simulink model "RigidbodyMPCCurvePathTracking"  (Simulink 9.3)
settings: Solver=ode45  StartTime=0.0  StopTime=38  FixedStep=0.01  RelTol=1e-3  EnableMultiTasking=on
libraries: Solver_SF x1
settings Model: Creator=xuwei  LastModifiedBy=梁秀华
settings DataIOCC: LimitDataPoints=on
settings OptimizationCC: ExpressionDepthLimit=2147483647
settings DebuggingCC: SolverPrmCheckMsg=warning  StateNameClashWarn=warning
settings GRTTargetCC: GeneratePreprocessorConditionals=Disable all

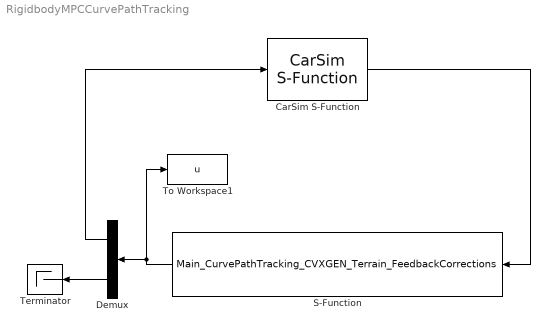
== system RigidbodyMPCCurvePathTracking ==
  CarSim S-Function : Solver_SF/CarSim S-Function  Priority=1  SIMFILE=simfile.sim
  Demux : Demux  Outputs=[1 14]
  S-Function : S-Function  FunctionName=Main_CurvePathTracking_CVXGEN_Terrain_FeedbackCorrections  SFunctionDeploymentMode=off  EnableBusSupport=off
  Terminator : Terminator
  To Workspace1 : ToWorkspace  VariableName=u  SaveFormat=Structure  SampleTime=-1
  wires:
  CarSim S-Function/1 -> S-Function/1
  S-Function/1 -> Demux/1, To Workspace1/1
  Demux/2 -> Terminator/1
  Demux/1 -> CarSim S-Function/1
